simulink model "My_AC"  (R2023a)
settings: Solver=VariableStepAuto  StartTime=0.0  StopTime=0.06  MaxStep=0.2e-6  RelTol=1e-3
libraries: spsMosfetLib x4, spsSeriesRLCBranchLib x3, spsMultimeterLib x2, spsACVoltageSourceLib x1, spsRMSLib x1, sps_lib x1
settings Model: Creator=张辉宇  LastModifiedBy=张辉宇
settings DataIOCC: ReturnWorkspaceOutputs=off

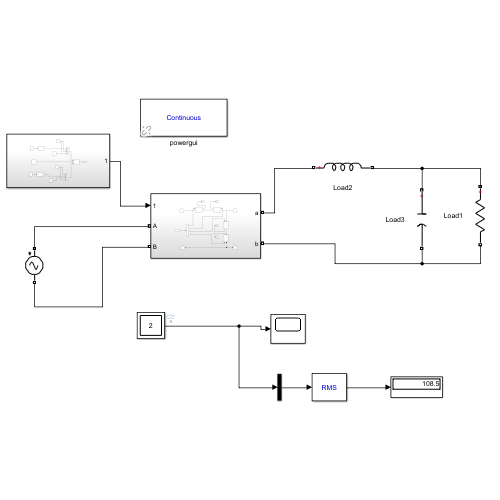
[thumbnail: Simulink's stored preview of the top-level diagram]
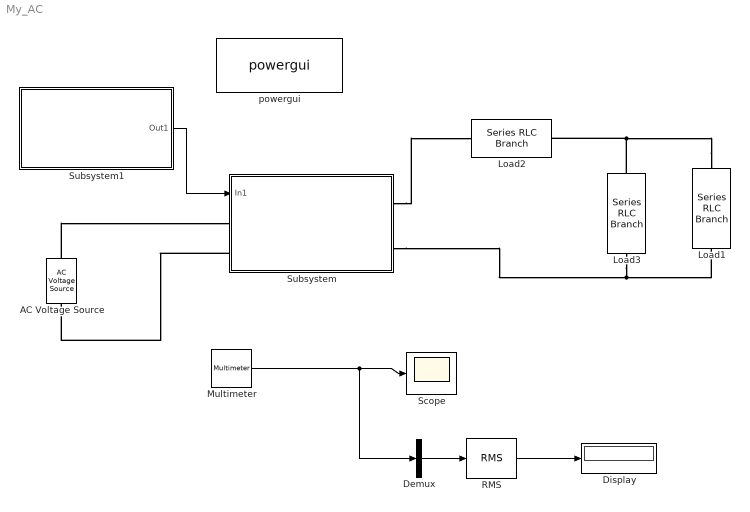
== system My_AC ==
  AC Voltage Source : spsACVoltageSourceLib/AC Voltage Source  Amplitude=220*sqrt(2)  Phase=0  Frequency=50  SampleTime=0  Measurements=Voltage  BusType=swing  Pref=10e3  Qref=0  Qmin=-inf  Qmax=+inf
  Demux : Demux  Outputs=1
  Display : Display
  Load1 : spsSeriesRLCBranchLib/Series RLC Branch  LConnTagsString=__new0  RConnTagsString=__new0  BranchType=R  Resistance=8  Inductance=1e-3  SetiL0=off  InitialCurrent=0  Capacitance=1e-6  Setx0=off  InitialVoltage=0  Measurements=Branch voltage and current
  Load2 : spsSeriesRLCBranchLib/Series RLC Branch  LConnTagsString=__new0  RConnTagsString=__new0  BranchType=L  Resistance=8  Inductance=1.2e-3  SetiL0=off  InitialCurrent=0  Capacitance=1e-6  Setx0=off  InitialVoltage=0  Measurements=None
  Load3 : spsSeriesRLCBranchLib/Series RLC Branch  LConnTagsString=__new0  RConnTagsString=__new0  BranchType=C  Resistance=8  Inductance=1e-3  SetiL0=off  InitialCurrent=0  Capacitance=1e-6  Setx0=off  InitialVoltage=0  Measurements=None
  Multimeter : spsMultimeterLib/Multimeter  L=3  sel=[1 3]  yselected={}  Gain=[1 1]  OutputType=Complex  PlotAtSimulationStop=off  PhasorSimulation=off
  RMS : spsRMSLib/RMS  TrueRMS=on  Freq=50  RMSInit=120  Ts=0
  Scope : Scope
  Subsystem : Subsystem
  Subsystem1 : Subsystem
  powergui : sps_lib/powergui  Priority=1  SimulationMode=Continuous  SampleTime=50e-6  frequency=60  Iterations=50  frequencyindice=50  Pbase=100e6  ErrMax=1e-4  UnitsV=kV  UnitsW=MW  buscounter=0  FunctionMessages=off  echomessages=off  EnableUseOfTLC=off  CurrentSourceSwitches=off  DisableSnubberDevices=off  DisableRonSwitches=off  DisableVfSwitches=off  DisplayEquations=off  AutomaticDiscreteSolvers=off  SolverType=Tustin/Backward Euler (TBE)  Interpol=off  ExternalGateDelay=off  methode=off  Ts=100  x0status=blocks  SPID=on  SwTol=0  HookPort=off  NonlinearTolerance=1e-4  nMaxIteration=100  ContinueOnMaxIteration=off  RestoreLinks=warning  ResistiveCurrentMeasurement=off  Frange=[0:2:500]  Ylog=off  Xlog=on  ShowGrid=off  save=off  variable=ZData  structure=0  ZoomFFT=off  StartTime=0.0  cycles=1  DisplayStyle=1  fundamental=60  FreqAxis=off  MaxFrequency=1000  frequencyindicesteady=1  RmsSteady=1  display=off
  wires:
  Multimeter/1 -> Demux/1, Scope/1
  Subsystem1/1(Out1) -> Subsystem/1(In1)
  Demux/1 -> RMS/1
  RMS/1 -> Display/1
  connections:
  AC Voltage Source/RConn1 -- Subsystem/LConn1
  Subsystem/LConn2 -- AC Voltage Source/LConn1
  Load1/LConn1 -- Load3/LConn1 -- Load2/RConn1
  Subsystem/RConn2 -- Load3/RConn1 -- Load1/RConn1
  Subsystem/RConn1 -- Load2/LConn1

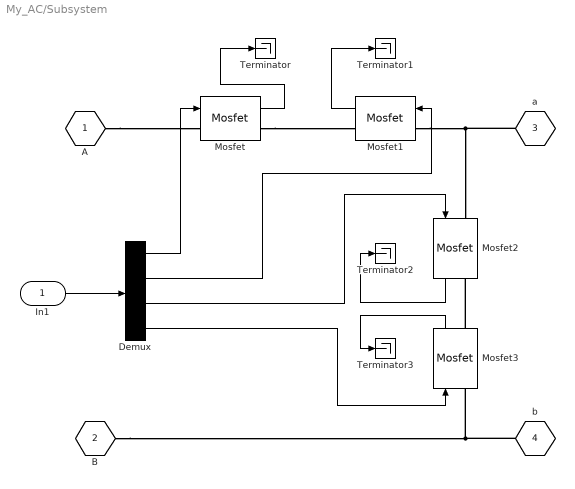
== system My_AC/Subsystem ==
  In1 : Inport
  Demux : Demux
  Mosfet{,1..3} (4 alike) : spsMosfetLib/Mosfet  Ron=0.1  Lon=0  Rd=0.01  Vfd=0  IC=0  Rs=1e5  Cs=inf  Measurements=on
  Terminator{,1..3} (4 alike) : Terminator
  A : PMIOPort  Side=Left
  B : PMIOPort  Port=2  Side=Left
  a : PMIOPort  Port=3  Side=Right
  b : PMIOPort  Port=4  Side=Right
  wires:
  In1/1 -> Demux/1
  Demux/1 -> Mosfet/1
  Demux/2 -> Mosfet1/1
  Demux/3 -> Mosfet2/1
  Demux/4 -> Mosfet3/1
  Mosfet/1 -> Terminator/1
  Mosfet1/1 -> Terminator1/1
  Mosfet2/1 -> Terminator2/1
  Mosfet3/1 -> Terminator3/1
  connections:
  Mosfet3/RConn1 -- Mosfet2/RConn1
  Mosfet1/LConn1 -- a/RConn1 -- Mosfet2/LConn1
  Mosfet/RConn1 -- Mosfet1/RConn1
  B/RConn1 -- b/RConn1 -- Mosfet3/LConn1
  A/RConn1 -- Mosfet/LConn1

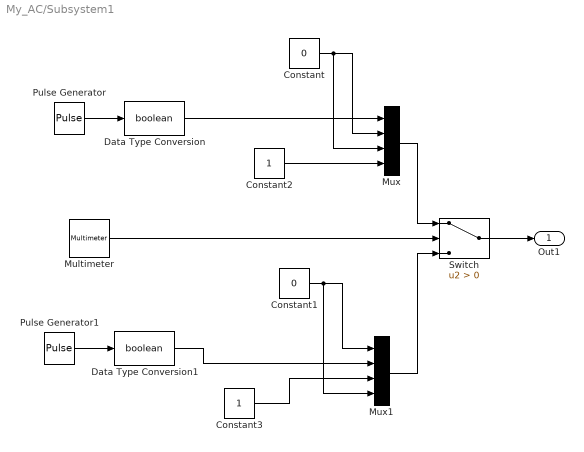
== system My_AC/Subsystem1 ==
  Constant : Constant  Value=0  OutDataTypeStr=boolean
  Constant1 : Constant  Value=0  OutDataTypeStr=boolean
  Constant2 : Constant  OutDataTypeStr=boolean
  Constant3 : Constant  OutDataTypeStr=boolean
  Data Type Conversion : DataTypeConversion  OutDataTypeStr=boolean  SaturateOnIntegerOverflow=off  RndMeth=Floor
  Data Type Conversion1 : DataTypeConversion  OutDataTypeStr=boolean  SaturateOnIntegerOverflow=off  RndMeth=Floor
  Multimeter : spsMultimeterLib/Multimeter  L=3  sel=2  yselected={}  Gain=1  OutputType=Complex  PlotAtSimulationStop=off  PhasorSimulation=off
  Mux : Mux
  Mux1 : Mux
  Pulse Generator : DiscretePulseGenerator  PulseType=Time based  Period=1/20e3  PulseWidth=50
  Pulse Generator1 : DiscretePulseGenerator  PulseType=Time based  Period=1/20e3  PulseWidth=50
  Switch : Switch  Criteria=u2 > Threshold  SaturateOnIntegerOverflow=off  InputSameDT=off
  Out1 : Outport
  wires:
  Multimeter/1 -> Switch/2
  Switch/1 -> Out1/1
  Pulse Generator/1 -> Data Type Conversion/1
  Data Type Conversion/1 -> Mux/1
  Constant/1 -> Mux/3, Mux/2
  Mux/1 -> Switch/1
  Data Type Conversion1/1 -> Mux1/2
  Pulse Generator1/1 -> Data Type Conversion1/1
  Constant1/1 -> Mux1/1, Mux1/4
  Mux1/1 -> Switch/3
  Constant2/1 -> Mux/4
  Constant3/1 -> Mux1/3
